simulink model "linePlan"  (R2020b)
settings: Solver=FixedStepAuto  StartTime=0.0  StopTime=inf  FixedStep=0.02  RelTol=1e-3
settings Model: Creator=GW00069596  LastModifiedBy=GW00216231
settings DataIOCC: ReturnWorkspaceOutputs=off
settings DebuggingCC: ArithmeticOperatorsInVariantConditions=warning
settings SFSimCC: SimUseLocalCustomCode=off  MATLABDynamicMemAlloc=off  CustomCodeUndefinedFunction=UseInterfaceOnly
settings RTWCC: RTWUseLocalCustomCode=off
settings CodeAppCC: StateflowObjectComments=on

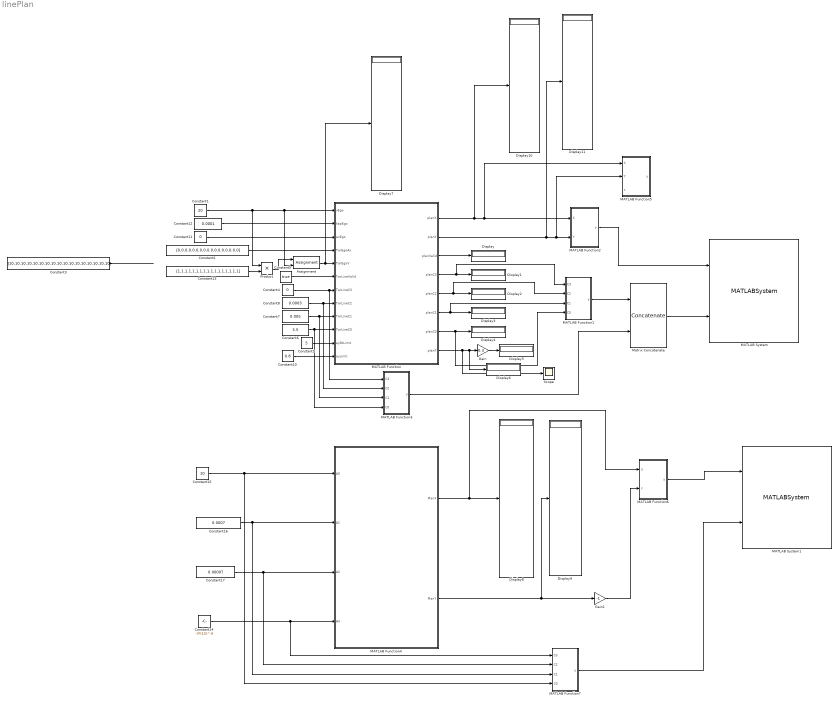
== system linePlan ==
  Assignment : Assignment  DiagnosticForDimensions=Warning  IndexOptions=Assign all  Indices=2  OutputSizes=1
  Constant1 : Constant  Value=20
  Constant10 : Constant  Value=0.8
  Constant11 : Constant  Value=0
  Constant12 : Constant  Value=0.0001
  Constant13 : Constant  Value=[1,1,1,1,1,1,1,1,1,1,1,1,1,1,1,1,1]
  Constant14 : Constant  Value=-3*(10)^-9
  Constant15 : Constant  Value=10
  Constant16 : Constant  Value=0.0007
  Constant17 : Constant  Value=0.00007
  Constant2 : Constant  Value=[0,0,0,0,0,0,0,0,0,0,0,0,0,0,0,0,0]
  Constant3 : Constant  Value=[10,10,10,10,10,10,10,10,10,10,10,10,10,10,10,10,10]
  Constant4 : Constant  Value=0
  Constant5 : Constant  Value=true
  Constant6 : Constant  Value=3.5
  Constant7 : Constant  Value=0.005
  Constant8 : Constant  Value=0.0003
  Constant9 : Constant  Value=5
  Display{,1..11} (12 alike) : Display
  Gain : Gain  Gain=0.3
  Gain1 : Gain  Gain=-1
  MATLAB Function : MATLAB Function  TreatAsAtomicUnit=on
  MATLAB Function1 : MATLAB Function  TreatAsAtomicUnit=on
  MATLAB Function2 : MATLAB Function  TreatAsAtomicUnit=on
  MATLAB Function3 : MATLAB Function  TreatAsAtomicUnit=on
  MATLAB Function4 : MATLAB Function  TreatAsAtomicUnit=on
  MATLAB Function5 : MATLAB Function  TreatAsAtomicUnit=on
  MATLAB Function6 : MATLAB Function  TreatAsAtomicUnit=on
  MATLAB Function7 : MATLAB Function  TreatAsAtomicUnit=on
  MATLAB System : MATLABSystem  System=BirdsEyeView17a  XLim=[ 0, 120 ]  YLim=[ -30, 30 ]  HasActors=off  ActorsColor=off  HasVision=off  HasRadar=on  HasRoads=on  HasLaneMarkings=off  Camera_Fov=52  Camera_Range=100  Camera_Yaw=0  Camera_Pos=[ 0, 0 ]  Radar_Fov=52  Radar_Range=100  Radar_Yaw=0  Radar_Pos=[ 0, 0 ]  MarkerSize=8  LabelFontSize=9  LabelOffset=[ 1.5, 1.5 ]  aspectratio=off
      mask Type: BirdsEyeView17a
      mask Display:
      | disp(['Bird''s-Eye' char(10) 'View']);
      | port_label('input',1,'Radar');
      | port_label('input',2,'Roads');
  MATLAB System1 : MATLABSystem  System=BirdsEyeView17a  XLim=[ 0, 120 ]  YLim=[ -30, 30 ]  HasActors=off  ActorsColor=off  HasVision=off  HasRadar=on  HasRoads=on  HasLaneMarkings=off  Camera_Fov=52  Camera_Range=100  Camera_Yaw=0  Camera_Pos=[ 0, 0 ]  Radar_Fov=52  Radar_Range=100  Radar_Yaw=0  Radar_Pos=[ 0, 0 ]  MarkerSize=8  LabelFontSize=9  LabelOffset=[ 1.5, 1.5 ]  aspectratio=off
      mask Type: BirdsEyeView17a
      mask Display:
      | disp(['Bird''s-Eye' char(10) 'View']);
      | port_label('input',1,'Radar');
      | port_label('input',2,'Roads');
  Matrix Concatenate : Concatenate  Mode=Multidimensional array
  Product : Product
  Scope : Scope
  wires:
  Constant2/1 -> MATLAB Function/4(TarEgoAx)
  Constant3/1 -> ?
  Constant5/1 -> MATLAB Function/6(TarLineValid)
  Constant4/1 -> MATLAB Function3/1(C3), MATLAB Function/7(TarLineC3)
  Constant6/1 -> MATLAB Function3/4(C0), MATLAB Function/10(TarLineC0)
  Constant7/1 -> MATLAB Function3/3(C1), MATLAB Function/9(TarLineC1)
  Constant8/1 -> MATLAB Function3/2(C2), MATLAB Function/8(TarLineC2)
  Constant9/1 -> MATLAB Function/11(ayDtLimit)
  MATLAB Function/3(planValid) -> Display/1
  MATLAB Function/4(planC3) -> MATLAB Function1/1(C3), Display1/1
  MATLAB Function/5(planC2) -> MATLAB Function1/2(C2), Display2/1
  MATLAB Function/6(planC1) -> MATLAB Function1/3(C1), Display3/1
  MATLAB Function/7(planC0) -> MATLAB Function1/4(C0), Display4/1
  MATLAB Function/8(planT) -> Display6/1, Gain/1, Scope/1
  Constant10/1 -> MATLAB Function/12(ayLimit)
  MATLAB Function1/1(y) -> Matrix Concatenate/1
  MATLAB Function/1(planX) -> Display10/1, MATLAB Function5/1(X), MATLAB Function2/1(X)
  MATLAB Function/2(planY) -> Display11/1, MATLAB Function5/2(Y), MATLAB Function2/2(Y)
  MATLAB Function2/1(y) -> MATLAB System/1
  Matrix Concatenate/1 -> MATLAB System/2
  MATLAB Function3/1(y) -> Matrix Concatenate/2
  Gain/1 -> Display5/1
  Constant1/1 -> Product/1, MATLAB Function/1(vEgo), Assignment/2
  Constant11/1 -> MATLAB Function/3(axEgo)
  Constant12/1 -> MATLAB Function/2(kapEgo)
  Assignment/1 -> Display7/1, MATLAB Function/5(TarEgoV)
  Constant13/1 -> Product/2
  Product/1 -> Assignment/1
  Constant15/1 -> MATLAB Function4/1(A0), MATLAB Function7/4(C0)
  Constant16/1 -> MATLAB Function7/3(C1), MATLAB Function4/2(A1)
  Constant17/1 -> MATLAB Function7/2(C2), MATLAB Function4/3(A2)
  Constant14/1 -> MATLAB Function7/1(C3), MATLAB Function4/4(A3)
  MATLAB Function4/1(PlanX) -> MATLAB Function6/1(X), Display8/1
  MATLAB Function4/2(PlanY) -> Gain1/1, Display9/1
  MATLAB Function6/1(y) -> MATLAB System1/1
  MATLAB Function7/1(y) -> MATLAB System1/2
  Gain1/1 -> MATLAB Function6/2(Y)

== matlab function linePlan/MATLAB Function7 ==
  data: C3 input; y output; C2 input; C1 input; C0 input
function y = line(C3,C2,C1,C0)

y = zeros(1,9);
y(1,1) = C3;
y(1,2) = C2;
y(1,3) = C1;
y(1,4) = C0;
y(1,5) = 0;
y(1,6) = 250;
y(1,7) = 0;
y(1,8) = 0;
y(1,9) = 1;

== matlab function linePlan/MATLAB Function1 ==
  data: C3 input; y output; C2 input; C1 input; C0 input
function y = line(C3,C2,C1,C0)

y = zeros(1,9);
y(1,1) = C3;
y(1,2) = C2;
y(1,3) = C1;
y(1,4) = C0;
y(1,5) = 0;
y(1,6) = 100;
y(1,7) = 0;
y(1,8) = 0;
y(1,9) = 1;

== matlab function linePlan/MATLAB Function ==
  data: planX output; planY output; vEgo input size=1; planValid output boolean size=1; kapEgo input size=1; axEgo input size=1; TarEgoAx input size=17; TarEgoV input size=17; TarLineValid input boolean size=1; TarLineC3 input size=1; TarLineC2 input size=1; TarLineC1 input size=1; TarLineC0 input size=1; ayDtLimit input size=1; ayLimit input size=1; planC3 output size=1; planC2 output size=1; planC1 output size=1; planC0 output size=1; planT output
function [planX,planY,planValid,planC3,planC2,planC1,planC0,planT] = ...
    linePlanCalc(vEgo,kapEgo,axEgo,TarEgoAx,TarEgoV,...
    TarLineValid,TarLineC3,TarLineC2,TarLineC1,TarLineC0,...
    ayDtLimit,ayLimit)

%    x(t) = a5*t^5 + a4*t^4 + a3*t^3 + a2*t^2 + a1*t + a0;
%    y(t) = b5*t^5 + b4*t^4 + b3*t^3 + b2*t^2 + b1*t + b0;
%    A = [a5;a4;a3;a2;a1;a0];
%    B = [b5;b4;b3;b2;b1;b0];

if TarLineValid
    if abs(TarLineC0)<0.15&&...
        abs(TarLineC1)<0.05
        planValid = true;
        planC3 = TarLineC3;
        planC2 = TarLineC2;
        planC1 = TarLineC1;
        planC0 = TarLineC0;
        planT = 11;
        planX = zeros(11,1);
        planY = zeros(11,1);
    else
        Px = 3:0.5:11;    % s
        if vEgo>1
            Px = vEgo*Px;
        end
        
        Py = TarLineC3*(Px.^3) + TarLineC2*(Px.^2) + TarLineC1*(Px.^1) + TarLineC0;
        
        
        x = zeros(11,1);
        y = zeros(11,1);
        Vx = zeros(11,1);
        Vy = zeros(11,1);
        Ax = zeros(11,1);
        Ay = zeros(11,1);
        AyDt = zeros(11,1);
        
        for i = 1:17
            Pt = 1.05*sqrt(Px(i)^2 + Py(i)^2)/max(1,0.5*(TarEgoV(i) + vEgo));
            t_Vego = max(vEgo,1);
            t0 = 0;
            tn = Pt;
            
            T = [t0^5,t0^4,t0^3,t0^2,t0,1;...
                5*t0^4,4*t0^3,3*t0^2,2*t0,1,0;...
                20*t0^3,12*t0^2,6*t0,2,0,0;...
                tn^5,tn^4,tn^3,tn^2,tn,1;...
                5*tn^4,4*tn^3,3*tn^2,2*tn,1,0;...
                20*tn^3,12*tn^2,6*tn,2,0,0];
            
            Vn = TarEgoV(i);
            An = TarEgoAx(i);
            kP =  3*TarLineC3*(Px(i).^2) + 2*TarLineC2*Px(i) + TarLineC1;
            Vxn = Vn/sqrt(1 + kP^2);
            Vyn = Vn*kP/sqrt(1 + kP^2);
            Axn = An/sqrt(1 + kP^2);
            Ayn = An*kP/sqrt(1 + kP^2);
            
            MaX = [0;t_Vego;axEgo;Px(i);Vxn;Axn];
            MaY = [0;0;(vEgo^2)*kapEgo;Py(i);Vyn;Ayn];
            A = T\MaX;
            B = T\MaY;
            
            a5 = A(1);
            a4 = A(2);
            a3 = A(3);
            a2 = A(4);
            a1 = A(5);
            a0 = A(6);
            
            b5 = B(1);
            b4 = B(2);
            b3 = B(3);
            b2 = B(4);
            b1 = B(5);
            b0 = B(6);
            
            preLineValid = true;
            for j=1:11
                t = (j-1)*tn/10;
                x(j) = a5*t^5 + a4*t^4 + a3*t^3 + a2*t^2 + a1*t + a0;
                Vx(j) = 5*a5*t^4 + 4*a4*t^3 + 3*a3*t^2 + 2*a2*t + a1;
                Ax(j) = 20*a5*t^3 + 12*a4*t^2 + 6*a3*t + 2*a2;
                y(j) = b5*t^5 + b4*t^4 + b3*t^3 + b2*t^2 + b1*t + b0;
                Vy(j) = 5*b5*t^4 + 4*b4*t^3 + 3*b3*t^2 + 2*b2*t + b1;
                Ay(j) = 20*b5*t^3 + 12*b4*t^2 + 6*b3*t + 2*b2;
                AyDt(j) = 60*b5*t^2 + 24*b4*t + 6*b3;
                if abs(Ay(j))>ayLimit||...
                        abs(AyDt(j))>ayDtLimit
                    preLineValid = false;
                    break;
                end
            end
            if preLineValid
                break;
            end
            if i == 17
                for j=1:11
                    t = (j-1)*tn/10;
                    x(j) = a5*t^5 + a4*t^4 + a3*t^3 + a2*t^2 + a1*t + a0;
                    Vx(j) = 5*a5*t^4 + 4*a4*t^3 + 3*a3*t^2 + 2*a2*t + a1;
                    Ax(j) = 20*a5*t^3 + 12*a4*t^2 + 6*a3*t + 2*a2;
                    y(j) = b5*t^5 + b4*t^4 + b3*t^3 + b2*t^2 + b1*t + b0;
                    Vy(j) = 5*b5*t^4 + 4*b4*t^3 + 3*b3*t^2 + 2*b2*t + b1;
                    Ay(j) = 20*b5*t^3 + 12*b4*t^2 + 6*b3*t + 2*b2;
                    AyDt(j) = 60*b5*t^2 + 24*b4*t + 6*b3;
                end
            end
        end
        
        % [planC3,planC2,planC1,planC0] = pl(x(1:4,1),y(1:4,1));
        xx1 = x(1,1);
        xx2 = x(4,1);
        xx3 = x(8,1);
        xx4 = x(11,1);
        xx = [xx1;xx2;xx3;xx4];
        yy1 = y(1,1);
        yy2 = y(4,1);
        yy3 = y(8,1);
        yy4 = y(11,1);
        yy = [yy1;yy2;yy3;yy4];
        [planC3,planC2,planC1,planC0] = pl(x(1:4,1),y(1:4,1));
        
        planValid = true;
        planT = Pt;
        planX = x;
        planY = y;
    end
else
    planValid = false;
    planC3 = 0;
    planC2 = 0;
    planC1 = 0;
    planC0 = 0;
    planT = 11;
    planX = zeros(11,1);
    planY = zeros(11,1);
end

== matlab function linePlan/MATLAB Function2 ==
  data: X input; y output; Y input
function y = line(X,Y)

y = zeros(11,8);
for i=1:11
    y(i,1) = X(i);
    y(i,2) = Y(i);
    y(i,3) = 1;
    y(i,4) = 0;
    y(i,5) = 0;
    y(i,6) = i;
    y(i,7) = 1;
    y(i,8) = 1;
end

== matlab function linePlan/MATLAB Function3 ==
  data: C3 input; y output; C2 input; C1 input; C0 input
function y = line(C3,C2,C1,C0)

y = zeros(1,9);
y(1,1) = C3;
y(1,2) = C2;
y(1,3) = C1;
y(1,4) = C0;
y(1,5) = 0;
y(1,6) = 250;
y(1,7) = 0;
y(1,8) = 0;
y(1,9) = 1;

== matlab function linePlan/MATLAB Function4 ==
  data: A0 input; A1 input; A2 input; A3 input; PlanX output size=[20,1]; PlanY output size=[20 1]
function [PlanX,PlanY]= fcn(A0,A1,A2,A3)
% 参考线离散化
rx1 = [single(0):single(1):single(9)];
rx2 = [single(10):20:150];
rx = cat(2,rx1,rx2);
ry = single((-1)).*(A0 + A1.* rx + A2.* (rx.^2) + A3.* (rx.^3));
waypoints = [ry',rx'];
referencePath = FrenentReferencePath(waypoints,5);
pathStart = referencePath.interpolate(0);% 求起始点处车辆状态 [x, y,theta, kappa, dkappa, s]
initialState=[0 -A0 pathStart(1,3)];

Frenet_traj_obj = TrajectoryGeneratorFrenet(referencePath,0.5);
arcLenOffsets = single(60);
ds = single(1);
[frenetTrajectory,globalTrajectory,numTraj] = Frenet_traj_obj.FrenetTrajectory_Lateral(initialState,arcLenOffsets,0,ds);
[globalTrajectory] = EvaluateTrajectory_Lateral(frenetTrajectory,globalTrajectory, 1,1)
% [s,d]→[x, y, theta, kappa, dkappa]
PlanX = single(zeros(20,1));
PlanY = single(zeros(20,1));
PlanX= globalTrajectory(1).Trajectory(1:20,2);
PlanY= globalTrajectory(1).Trajectory(1:20,1);
end

== matlab function linePlan/MATLAB Function5 ==
  data: X input; y output; Y input; x input
function y = line(X,Y,x)
y =interp1(X,Y,x,'linear');
end

== matlab function linePlan/MATLAB Function6 ==
  data: X input; y output; Y input
function y = line(X,Y)

y = zeros(20,8);
for i=1:20
    y(i,1) = X(i);
    y(i,2) = Y(i);
    y(i,3) = 1;
    y(i,4) = 0;
    y(i,5) = 0;
    y(i,6) = i;
    y(i,7) = 1;
    y(i,8) = 1;
end
